simulink model "AD_stepper_simulation_all"  (Simulink 10.0)
settings: Solver=ode45  StartTime=0.0  StopTime=10  RelTol=1e-4  EnableMultiTasking=on
PostLoadFcn:
  | AD_stepper_parameter;
  | Ts = 0.01;     % sample time
  | Tmax = 0.5;  % maximum duration of a pulse
libraries: AD_Stepper_motor_lib x3
settings Model: Creator=qtian  LastModifiedBy=bhisma
settings DataIOCC: LimitDataPoints=on  SignalLoggingSaveFormat=ModelDataLogs
settings OptimizationCC: BlockReduction=off  OptimizeBlockIOStorage=off  BufferReuse=off  GlobalBufferReuse=off  ExpressionFolding=off  ExpressionDepthLimit=2147483647  LocalBlockOutputs=off  InitFltsAndDblsToZero=on  OptimizeDataStoreBuffers=off  BusAssignmentInplaceUpdate=off
settings DebuggingCC: SaveWithParameterizedLinksMsg=none  SignalResolutionControl=TryResolveAllWithWarning  SolverPrmCheckMsg=warning  MultiTaskDSMMsg=warning  MultiTaskCondExecSysMsg=none  FcnCallInpInsideContextMsg=warning  StateNameClashWarn=warning
settings HardwareCC: ProdIntDivRoundTo=Zero  ProdEndianess=BigEndian  ProdHWDeviceType=Specified  TargetIntDivRoundTo=Zero  TargetEndianess=BigEndian
settings GRTTargetCC: GeneratePreprocessorConditionals=Disable all
settings ConfigComp: CovExternalEMLEnable=off

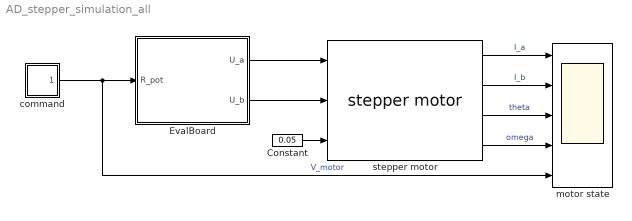
== system AD_stepper_simulation_all ==
  Constant : Constant  Value=0.05
  EvalBoard : Subsystem  TreatAsAtomicUnit=on  SystemSampleTime=Ts
  command : Subsystem  mask(Repeating table){rep_seq_t=[0:10], rep_seq_y=[0 0 -0.8 -0.8 0 0 0.5 0.9 0.8 0.2 0]}
      mask prompts: rep_seq_t "Time values:"; rep_seq_y "Output values:"
      mask help: Output a repeating sequence of numbers specified in a table of time-value pairs. Values of time should be monotonically increasing.
      mask init:
      | if (length(rep_seq_t) ~= length(rep_seq_y)),
      |   error('Length of time vector and output vector must be the same.')
      | end
      | dbl_rep_seq_t = double(rep_seq_t);
      | dbl_rep_seq_y = double(rep_seq_y);
      | period = max(dbl_rep_seq_t) - min(dbl_rep_seq_t);
      | period = str2num(sprintf('%0.5g',period));
      | s = round(length(dbl_rep_seq_t)/50);
      | if s > 0
      |   pts = [1:s:length(dbl_rep_seq_t)];
      |   L   = length(pts);
      | else
      |   L   = length(dbl_rep_seq_t);
      |   pts = [1:L];
      | end
      | 
      | disp_seq_t = reshape(dbl_rep_seq_t(pts),L,1);
      | disp_seq_y = reshape(dbl_rep_seq_y(pts),L,1);
      | disp_period = max(disp_seq_t) - min(disp_seq_t);
      | 
      | disp_seq_t  = repmat(disp_seq_t,1,3) + (ones(L,1)*(disp_period*[0,1,2]));
      | disp_seq_t = [ disp_seq_t(:); disp_seq_t(end) ];
      | disp_seq_y = repmat(disp_seq_y,1,3);
      | disp_seq_y = [ disp_seq_y(:); disp_seq_y(1) ];
      mask Help: Repeats cycle given in table. Time values should be monotonically increasing.
      mask Display: plot( disp_seq_t, disp_seq_y )
  motor state : Scope  NumInputPorts=5
  stepper motor : AD_Stepper_motor_lib/stepper motor  SystemSampleTime=-1
  wires:
  Constant/1 -> stepper motor/3
  stepper motor/1 -> motor state/1  "I_a"
  stepper motor/2 -> motor state/2  "I_b"
  EvalBoard/1(U_a) -> stepper motor/1
  EvalBoard/2(U_b) -> stepper motor/2
  command/1(Out1) -> EvalBoard/1(R_pot), motor state/5  "V_motor"
  stepper motor/3 -> motor state/3  "theta"
  stepper motor/4 -> motor state/4  "omega"

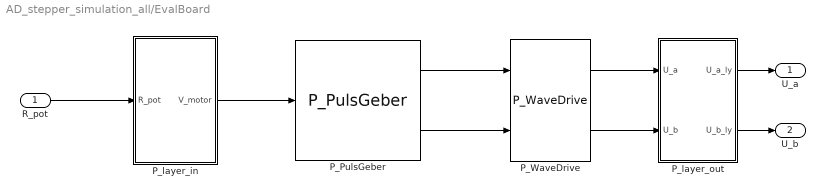
== system AD_stepper_simulation_all/EvalBoard ==
  R_pot : Inport
  P_PulsGeber : AD_Stepper_motor_lib/P_PulsGeber  SystemSampleTime=Ts
  P_WaveDrive : AD_Stepper_motor_lib/P_WaveDrive  SystemSampleTime=Ts
  P_layer_in : Subsystem  TreatAsAtomicUnit=on
  P_layer_out : Subsystem  TreatAsAtomicUnit=on  SystemSampleTime=Ts
  U_a : Outport
  U_b : Outport  Port=2
  wires:
  P_PulsGeber/1 -> P_WaveDrive/1
  P_PulsGeber/2 -> P_WaveDrive/2
  P_layer_out/1(U_a_ly) -> U_a/1
  P_layer_out/2(U_b_ly) -> U_b/1
  P_layer_in/1(V_motor) -> P_PulsGeber/1
  P_WaveDrive/1 -> P_layer_out/1(U_a)
  P_WaveDrive/2 -> P_layer_out/2(U_b)
  R_pot/1 -> P_layer_in/1(R_pot)

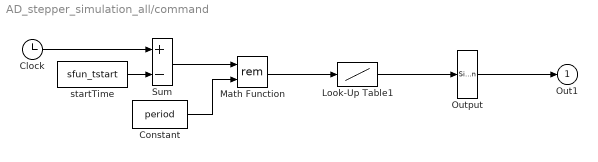
== system AD_stepper_simulation_all/command ==
  Clock : Clock
      settings: DisableCoverage=on
  Constant : Constant  DisableCoverage=on  Value=period
  Look-Up Table1 : Lookup  DisableCoverage=on  InputValues=rep_seq_t - min(rep_seq_t)  Table=rep_seq_y  SaturateOnIntegerOverflow=on
  Math Function : Math  DisableCoverage=on  Operator=rem  SaturateOnIntegerOverflow=on
  Output : SignalConversion  ConversionOutput=Contiguous copy  OverrideOpt=off
  Sum : Sum  DisableCoverage=on  Inputs=+-  SaturateOnIntegerOverflow=on  InputSameDT=on  OutDataTypeStr=Inherit: Same as first input
  startTime : S-Function  DisableCoverage=on  FunctionName=sfun_tstart  SFunctionDeploymentMode=off  EnableBusSupport=off
  Out1 : Outport
  wires:
  Constant/1 -> Math Function/2
  Output/1 -> Out1/1
  Look-Up Table1/1 -> Output/1
  startTime/1 -> Sum/2
  Clock/1 -> Sum/1
  Sum/1 -> Math Function/1
  Math Function/1 -> Look-Up Table1/1

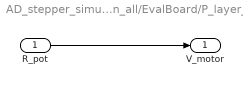
== system AD_stepper_simulation_all/EvalBoard/P_layer_in ==
  R_pot : Inport
  V_motor : Outport
  wires:
  R_pot/1 -> V_motor/1

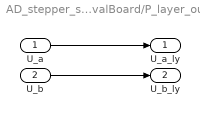
== system AD_stepper_simulation_all/EvalBoard/P_layer_out ==
  U_a : Inport
  U_b : Inport  Port=2
  U_a_ly : Outport
  U_b_ly : Outport  Port=2
  wires:
  U_a/1 -> U_a_ly/1
  U_b/1 -> U_b_ly/1
